simulink model "sim3d_surround_harness"  (R2025b)
settings: Solver=FixedStepAuto  StartTime=0.0  StopTime=10.0  FixedStep=1/60  RelTol=1e-3
libraries: sim3dcameralib x4, sim3dautolib x1, sim3dlib x1
settings Model: Creator=SAHIL  LastModifiedBy=SAHIL

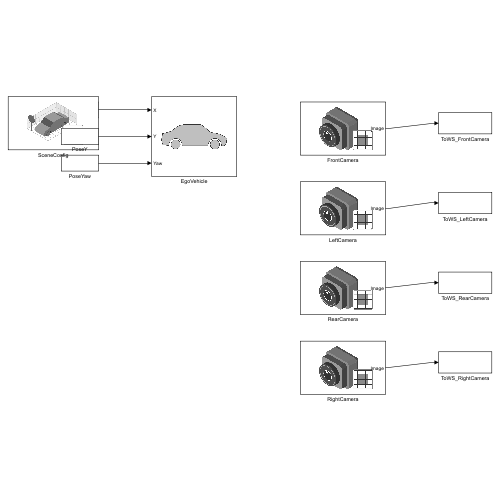
[thumbnail: Simulink's stored preview of the top-level diagram]
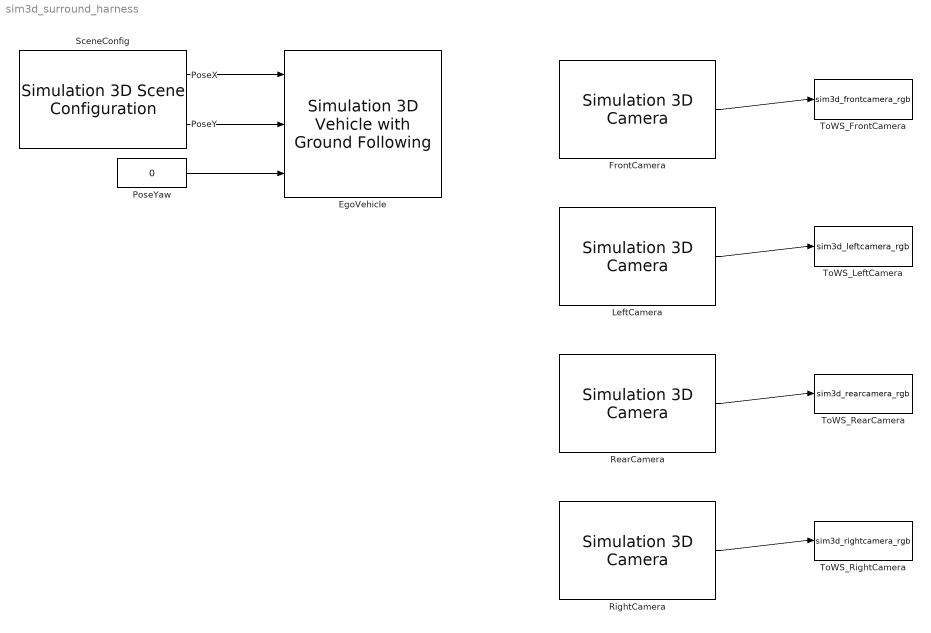
== system sim3d_surround_harness ==
  EgoVehicle : sim3dautolib/Simulation 3D Vehicle with Ground Following  Priority=-1  PassVehMesh=Muscle car  MeshPath=/MathWorksAutomotiveContent/Vehicles/Muscle/Meshes/SK_MuscleCar.SK_MuscleCar  TrackWidth=1.9  WheelBase=3  WheelRadius=0.35  VehColor=Red  CoordinateSystem=ISO8855  InitialPos=[0, 0, 0]  InitialRot=[0, 0, 0]  ActorName=SimulinkVehicle1  SampleTime=-1  ActorType=SimulinkVehicle  ID=1  aMode=3  ActorTag=Sim3DVehicle1  CoordinateScheme=0  VehLightsControl=off  HeadlightColor=[ 1, 1, 1 ]  HighBeamIntensity=100000  LowBeamIntensity=60000  HighBeamConeAngle=70  LowBeamConeAngle=70  LeftHeadlightOrientation=[ 0, 0 ]  RightHeadlightOrientation=[ 0, 0 ]  BrakelightIntensity=500  ReverselightIntensity=500  SignallightIntensity=500  SignallightPeriod=1  SignalPulseWidth=50  TransformOutportEnabled=off
      settings: LibrarySourceBlock=drivingsim3d/Simulation 3D Vehicle with Ground Following
  FrontCamera : sim3dcameralib/Simulation 3D Camera  Priority=1  sensorTag=Sim3dSensor  sensorId=1  sensorName=Sim3dSensor  vehTagList={'Scene Origin';'SimulinkVehicle1'}  vehTag=SimulinkVehicle1  CoordinateSystem=ISO8855  mountLoc=Origin  offsetFlag=off  tmountOffset=[2.2 0.0 1.35]  extTmount=off  rmountOffset=[0 6 0]  extRmount=off  FocalLength=[1109, 1109]  OpticalCenter=[640, 360]  ImageSize=[720 1280]  RadialDistortion=[0, 0]  TangentialDistortion=[0, 0]  SensorSkew=0  VisualizeFieldOfView=off  FieldOfViewRange=61  DepthOutportEnabled=off  SemanticOutportEnabled=off  TransformOutportEnabled=off  SampleTime=30/60  mountPoint=[0 0 0]  mountOrientation=[0 0 0]  aMode=3  ID=1
      settings: LibrarySourceBlock=drivingsim3d/Simulation 3D Camera
  LeftCamera : sim3dcameralib/Simulation 3D Camera  Priority=1  sensorTag=Sim3dSensor  sensorId=2  sensorName=Sim3dSensor  vehTagList={'Scene Origin';'SimulinkVehicle1'}  vehTag=SimulinkVehicle1  CoordinateSystem=ISO8855  mountLoc=Origin  offsetFlag=off  tmountOffset=[0.8 1.05 1.20]  extTmount=off  rmountOffset=[0 8 90]  extRmount=off  FocalLength=[1109, 1109]  OpticalCenter=[640, 360]  ImageSize=[720 1280]  RadialDistortion=[0, 0]  TangentialDistortion=[0, 0]  SensorSkew=0  VisualizeFieldOfView=off  FieldOfViewRange=61  DepthOutportEnabled=off  SemanticOutportEnabled=off  TransformOutportEnabled=off  SampleTime=30/60  mountPoint=[0 0 0]  mountOrientation=[0 0 0]  aMode=3  ID=2
      settings: LibrarySourceBlock=drivingsim3d/Simulation 3D Camera
  PoseX : Constant  Value=0
  PoseY : Constant  Value=0
  PoseYaw : Constant  Value=0
  RearCamera : sim3dcameralib/Simulation 3D Camera  Priority=1  sensorTag=Sim3dSensor  sensorId=3  sensorName=Sim3dSensor  vehTagList={'Scene Origin';'SimulinkVehicle1'}  vehTag=SimulinkVehicle1  CoordinateSystem=ISO8855  mountLoc=Origin  offsetFlag=off  tmountOffset=[-2.2 0.0 1.15]  extTmount=off  rmountOffset=[0 8 180]  extRmount=off  FocalLength=[1109, 1109]  OpticalCenter=[640, 360]  ImageSize=[720 1280]  RadialDistortion=[0, 0]  TangentialDistortion=[0, 0]  SensorSkew=0  VisualizeFieldOfView=off  FieldOfViewRange=61  DepthOutportEnabled=off  SemanticOutportEnabled=off  TransformOutportEnabled=off  SampleTime=30/60  mountPoint=[0 0 0]  mountOrientation=[0 0 0]  aMode=3  ID=3
      settings: LibrarySourceBlock=drivingsim3d/Simulation 3D Camera
  RightCamera : sim3dcameralib/Simulation 3D Camera  Priority=1  sensorTag=Sim3dSensor  sensorId=4  sensorName=Sim3dSensor  vehTagList={'Scene Origin';'SimulinkVehicle1'}  vehTag=SimulinkVehicle1  CoordinateSystem=ISO8855  mountLoc=Origin  offsetFlag=off  tmountOffset=[0.8 -1.05 1.20]  extTmount=off  rmountOffset=[0 8 -90]  extRmount=off  FocalLength=[1109, 1109]  OpticalCenter=[640, 360]  ImageSize=[720 1280]  RadialDistortion=[0, 0]  TangentialDistortion=[0, 0]  SensorSkew=0  VisualizeFieldOfView=off  FieldOfViewRange=61  DepthOutportEnabled=off  SemanticOutportEnabled=off  TransformOutportEnabled=off  SampleTime=30/60  mountPoint=[0 0 0]  mountOrientation=[0 0 0]  aMode=3  ID=4
      settings: LibrarySourceBlock=drivingsim3d/Simulation 3D Camera
  SceneConfig : sim3dlib/Simulation 3D Scene Configuration  Priority=0  ProjectFormat=Default Scenes  SceneDesc=Straight road  ProjectName=E:\Program Files\MATLAB\R2025b\toolbox\shared\sim3d_projects\automotive_project_windows\UE\WindowsNoEditor\VehicleSimulation.exe  ScenePath=/Game/Maps/HwStrght  EnableOpenDRIVE=off  vehTagList={'Custom';'Scene Origin'}  vehTag=Scene Origin  AttachedCameraRelativeTranslation=[0 0 0]  FreeCameraDefaultInitialTranslation=[-6, 0, 2]  AttachedCameraRelativeRotation=[0 0 0]  FreeCameraDefaultInitialRotation=[0, -15, 0]  ViewpointName=Custom  FreeCameraInitialTranslation=[0, 0, 0]  ViewpointTranslation=[0 0 0]  FreeCameraInitialRotation=[0, 0, 0]  ViewpointRotation=[0 0 0]  OpVisEn=off  Ts=1/60  EnableWindow=on  EnableRemoteAccess=off  EnableWeather=off  SunAzimuth=90  SunAltitude=40.0  EnableGeospatialSun=off  Latitude=0  Longitude=0  Date=2023-01-01  Time=10:30:00  GeoTimeZone=-5.0  SunDaylightSaving=off  wind=1  clouds=10  EnableVolumetricClouds=off  CloudCoverage=0  CloudAltitude=6  fog=0  rain=0  RaindropsEffect=off  SnowDensity=0  EnableGeospatial=off  TilesetSource=Earth terrain  UseTrueOrigin=off  OriginHeight=200  OriginLatitude=40.744652  OriginLongitude=-73.988864  MapStyle=Aerial  AdditionalAssetIDs=[]  UseAdvancedSunSky=off  SolarTime=11  TimeZone=-5  Day=21  Month=9  Year=2022  UseDaylightSavingTime=on  DSTStartDay=10  DSTStartMonth=3  DSTEndDay=3  DSTEndMonth=11  DSTSwitchHour=2  sensorTag=MainCamera1  sensorId=1  sensorName=MainCamera1  mountLoc=Origin  offsetFlag=off  tmountOffset=[0, 0, 0]  rmountOffset=[0, 0, 0]  HorizontalResolution=1280  VerticalResolution=720  HorizontalFOV=60  mountPoint=[0 0 0]  mountOrientation=[0 0 0]  aMode=3  ID=1  GeoTrigger=Inactive  ViewNameList={'Custom'}  ViewTranslationList={'[0 0 0]'}  ViewRotationList={'[0 0 0]'}
      settings: LibrarySourceBlock=drivingsim3d/Simulation 3D Scene Configuration
  ToWS_FrontCamera : ToWorkspace  VariableName=sim3d_frontcamera_rgb  SaveFormat=Timeseries  SampleTime=-1
  ToWS_LeftCamera : ToWorkspace  VariableName=sim3d_leftcamera_rgb  SaveFormat=Timeseries  SampleTime=-1
  ToWS_RearCamera : ToWorkspace  VariableName=sim3d_rearcamera_rgb  SaveFormat=Timeseries  SampleTime=-1
  ToWS_RightCamera : ToWorkspace  VariableName=sim3d_rightcamera_rgb  SaveFormat=Timeseries  SampleTime=-1
  wires:
  PoseX/1 -> EgoVehicle/1
  PoseY/1 -> EgoVehicle/2
  PoseYaw/1 -> EgoVehicle/3
  FrontCamera/1 -> ToWS_FrontCamera/1
  LeftCamera/1 -> ToWS_LeftCamera/1
  RearCamera/1 -> ToWS_RearCamera/1
  RightCamera/1 -> ToWS_RightCamera/1
